simulink model "ident_posdcmotor"  (R2017a)
settings: Solver=FixedStepAuto  StartTime=0.0  StopTime=inf  RelTol=1e-3  EnableMultiTasking=on
undefined symbols (not defined in the file): DiscIntNeverNeededParam
libraries: arduinolib x3, simulink x2
settings Model: SimulationMode=external  ExtModeTrigDuration=2  Creator=Caue  LastModifiedBy=Caue
settings OptimizationCC: PassReuseOutputArgsAs=Individual arguments  MaxStackSize=64
settings DebuggingCC: ParameterTunabilityLossMsg=error
settings HardwareCC: ProdBitPerInt=16  ProdBitPerPointer=16  ProdBitPerSizeT=16  ProdBitPerPtrDiffT=16  ProdLargestAtomicFloat=None  ProdWordSize=8  ProdHWDeviceType=Atmel->AVR
settings SFSimCC: MATLABDynamicMemAlloc=off
settings RTWCC: SystemTargetFile=ert.tlc  HardwareBoard=Arduino Uno  TLCOptions=-aInlineSetEventsForThisBaseRateFcn=TLC_FALSE -aSuppressMultiTaskScheduler=TLC_FALSE -aRateBasedStepFcn=1  TemplateMakefile=ert_default_tmf  Description=Embedded Coder  GenerateReport=on  Toolchain=Arduino AVR  BuildConfiguration=Faster Runs  IncludeHyperlinkInReport=on  LaunchReport=on  GenerateTraceInfo=on  GenerateTraceReport=on  GenerateTraceReportSl=on  GenerateTraceReportSf=on  GenerateTraceReportEml=on
settings CodeAppCC: ForceParamTrailComments=on  IgnoreCustomStorageClasses=off  OperatorAnnotations=on  SimulinkDataObjDesc=on  SFDataObjDesc=on  MATLABFcnDesc=on  InsertBlockDesc=on  MATLABSourceComments=on
settings ERTTargetCC: SupportContinuousTime=on  SupportVariableSizeSignals=on

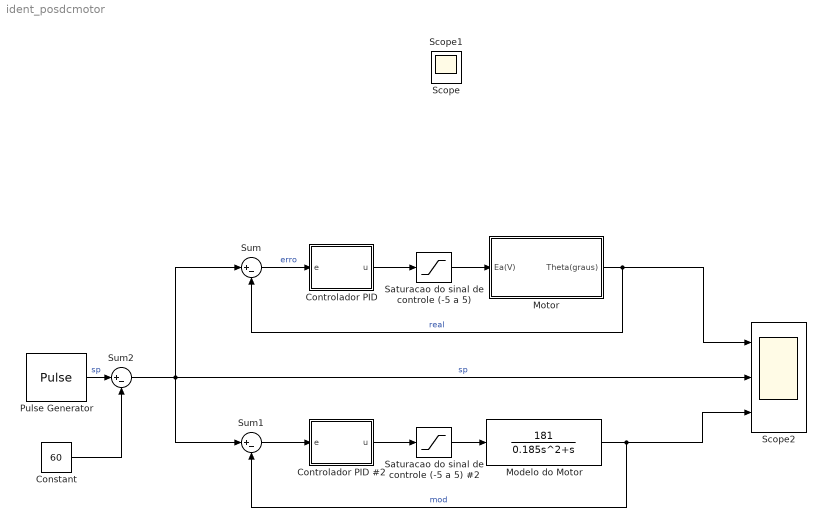
== system ident_posdcmotor ==
  Constant : Constant  Value=60
  Controlador PID : Subsystem  mask{Kp=0.1, Kd=0.0, Ki=0.0}
  Controlador PID #2 : Subsystem  mask{Kp=0.1, Kd=0.0, Ki=0.0}
  Modelo do Motor : TransferFcn  Numerator=[181]  Denominator=[0.185 1 0]
  Motor : Subsystem
  Pulse Generator : DiscretePulseGenerator  Amplitude=120  Period=10/0.02  PulseWidth=10/0.02/2  SampleTime=0.01
  Saturacao do sinal de controle (-5 a 5) : Saturate  UpperLimit=5  LowerLimit=-5
  Saturacao do sinal de controle (-5 a 5) #2 : Saturate  UpperLimit=5  LowerLimit=-5
  Scope2 : Scope  NumInputPorts=3
  Sum : Sum  Inputs=|+-
  Sum1 : Sum  Inputs=|+-
  Sum2 : Sum  Inputs=|+-
  Scope : Scope
  Scope1 : Scope
  wires:
  Motor/1(Theta(graus)) -> Sum/2, Scope2/1  "real"
  Sum2/1 -> Sum1/1, Scope2/2, Sum/1  "sp"
  Saturacao do sinal de controle (-5 a 5)/1 -> Motor/1(Ea(V))
  Sum/1 -> Controlador PID/1(e)  "erro"
  Controlador PID/1(u) -> Saturacao do sinal de controle (-5 a 5)/1
  Controlador PID #2/1(u) -> Saturacao do sinal de controle (-5 a 5) #2/1
  Sum1/1 -> Controlador PID #2/1(e)
  Saturacao do sinal de controle (-5 a 5) #2/1 -> Modelo do Motor/1
  Modelo do Motor/1 -> Scope2/3, Sum1/2  "mod"
  Pulse Generator/1 -> Sum2/1  "sp"
  Constant/1 -> Sum2/2

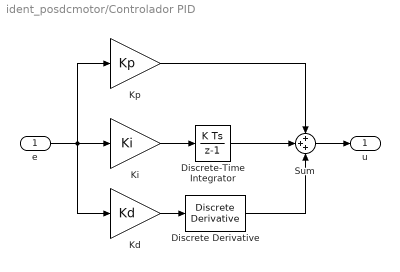
== system ident_posdcmotor/Controlador PID ==
  e : Inport
  Discrete Derivative : simulink/Discrete/Discrete Derivative  gainval=1.0  ICPrevScaledInput=0.0  OutMin=[]  OutMax=[]  OutDataType=fixdt(1, 16)  OutScaling=2^-10  DoSatur=off
  Discrete-Time Integrator : DiscreteIntegrator  InitialConditionSetting=State (most efficient)  SampleTime=-1  ICPrevOutput=DiscIntNeverNeededParam  ICPrevScaledInput=DiscIntNeverNeededParam
  Kd : Gain  Gain=Kd
  Ki : Gain  Gain=Ki
  Kp : Gain  Gain=Kp
  Sum : Sum  Inputs=+++
  u : Outport
  wires:
  e/1 -> Kp/1, Kd/1, Ki/1
  Ki/1 -> Discrete-Time Integrator/1
  Kd/1 -> Discrete Derivative/1
  Sum/1 -> u/1
  Discrete-Time Integrator/1 -> Sum/2
  Kp/1 -> Sum/1
  Discrete Derivative/1 -> Sum/3

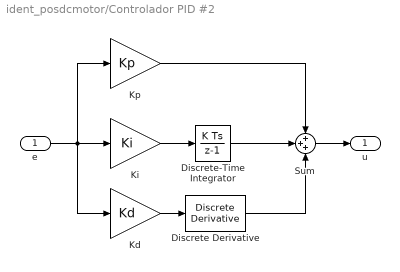
== system ident_posdcmotor/Controlador PID #2 ==
  e : Inport
  Discrete Derivative : simulink/Discrete/Discrete Derivative  gainval=1.0  ICPrevScaledInput=0.0  OutMin=[]  OutMax=[]  OutDataType=fixdt(1, 16)  OutScaling=2^-10  DoSatur=off
  Discrete-Time Integrator : DiscreteIntegrator  InitialConditionSetting=State (most efficient)  SampleTime=-1  ICPrevOutput=DiscIntNeverNeededParam  ICPrevScaledInput=DiscIntNeverNeededParam
  Kd : Gain  Gain=Kd
  Ki : Gain  Gain=Ki
  Kp : Gain  Gain=Kp
  Sum : Sum  Inputs=+++
  u : Outport
  wires:
  Discrete Derivative/1 -> Sum/3
  Kp/1 -> Sum/1
  Discrete-Time Integrator/1 -> Sum/2
  Sum/1 -> u/1
  Kd/1 -> Discrete Derivative/1
  Ki/1 -> Discrete-Time Integrator/1
  e/1 -> Ki/1, Kd/1, Kp/1

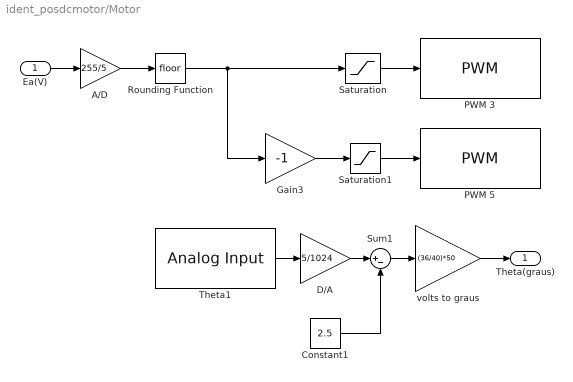
== system ident_posdcmotor/Motor ==
  Ea(V) : Inport
  A/D : Gain  Gain=255/5
  Constant1 : Constant  Value=2.5
  D/A : Gain  Gain=5/1024
  Gain3 : Gain  Gain=-1
  PWM 3 : arduinolib/PWM  pinNumber=3  blockPlatform=arduino
  PWM 5 : arduinolib/PWM  pinNumber=5  blockPlatform=arduino
  Rounding Function : Rounding
  Saturation : Saturate  UpperLimit=255  LowerLimit=0
  Saturation1 : Saturate  UpperLimit=255  LowerLimit=0
  Sum1 : Sum  Inputs=|+-
  Theta1 : arduinolib/Analog Input  pinNumber=1  sampleTime=0.01  blockPlatform=arduino
  volts to graus : Gain  Gain=(36/40)*50
  Theta(graus) : Outport
  wires:
  A/D/1 -> Rounding Function/1
  Gain3/1 -> Saturation1/1
  Saturation/1 -> PWM 3/1
  Rounding Function/1 -> Gain3/1, Saturation/1
  D/A/1 -> Sum1/1
  Sum1/1 -> volts to graus/1
  volts to graus/1 -> Theta(graus)/1
  Constant1/1 -> Sum1/2
  Saturation1/1 -> PWM 5/1
  Theta1/1 -> D/A/1
  Ea(V)/1 -> A/D/1
